simulink model "SimonPablobej3simul"  (R2018a)
settings: Solver=VariableStepAuto  StartTime=0.0  StopTime=10.0  RelTol=1e-3
settings Model: Creator=simon.suarez  LastModifiedBy=simon.suarez

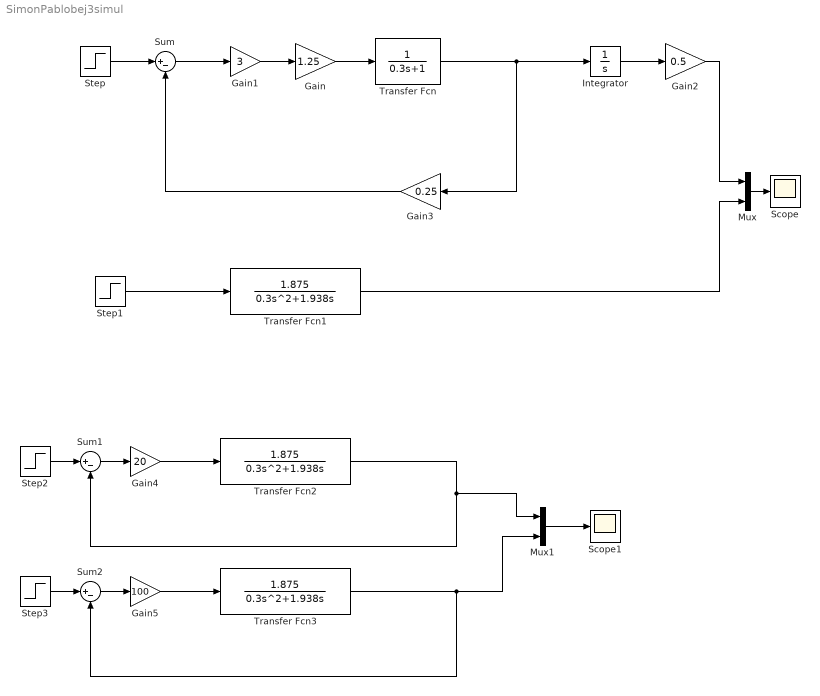
== system SimonPablobej3simul ==
  Gain : Gain  Gain=1.25
  Gain1 : Gain  Gain=3
  Gain2 : Gain  Gain=0.5
  Gain3 : Gain  Gain=0.25
  Gain4 : Gain  Gain=20
  Gain5 : Gain  Gain=100
  Integrator : Integrator
  Mux : Mux  Inputs=2
  Mux1 : Mux  Inputs=2
  Scope : Scope
  Scope1 : Scope
  Step{,1..3} (4 alike) : Step  SampleTime=0
  Sum : Sum  Inputs=|+-
  Sum1 : Sum  Inputs=|+-
  Sum2 : Sum  Inputs=|+-
  Transfer Fcn : TransferFcn  Denominator=[0.3 1]
  Transfer Fcn1 : TransferFcn  Numerator=[1.875]  Denominator=[0.3 1.938 0]
  Transfer Fcn2 : TransferFcn  Numerator=[1.875]  Denominator=[0.3 1.938 0]
  Transfer Fcn3 : TransferFcn  Numerator=[1.875]  Denominator=[0.3 1.938 0]
  wires:
  Gain1/1 -> Gain/1
  Gain/1 -> Transfer Fcn/1
  Transfer Fcn/1 -> Gain3/1, Integrator/1
  Integrator/1 -> Gain2/1
  Gain2/1 -> Mux/1
  Gain3/1 -> Sum/2
  Sum/1 -> Gain1/1
  Step/1 -> Sum/1
  Step1/1 -> Transfer Fcn1/1
  Transfer Fcn1/1 -> Mux/2
  Mux/1 -> Scope/1
  Gain4/1 -> Transfer Fcn2/1
  Step2/1 -> Sum1/1
  Sum1/1 -> Gain4/1
  Transfer Fcn2/1 -> Mux1/1, Sum1/2
  Transfer Fcn3/1 -> Mux1/2, Sum2/2
  Step3/1 -> Sum2/1
  Sum2/1 -> Gain5/1
  Gain5/1 -> Transfer Fcn3/1
  Mux1/1 -> Scope1/1
